simulink model "phase1_baseline"  (R2026a)
settings: Solver=VariableStepAuto
model workspace (MAT data in the model file):
  tau = 0
undefined symbols (not defined in the file): actuationDelay_s, simulationParams
settings Model: Creator=rayyu  LastModifiedBy=rayyu

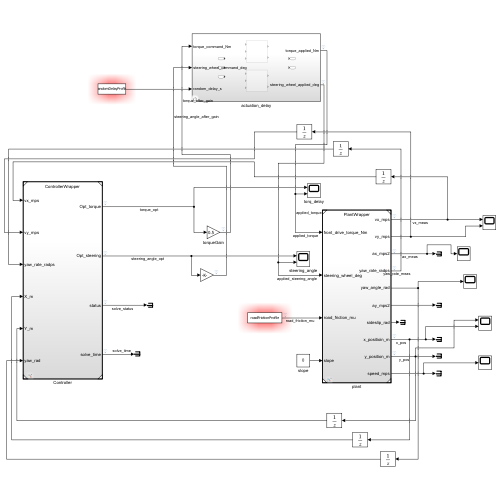
[thumbnail: Simulink's stored preview of the top-level diagram]
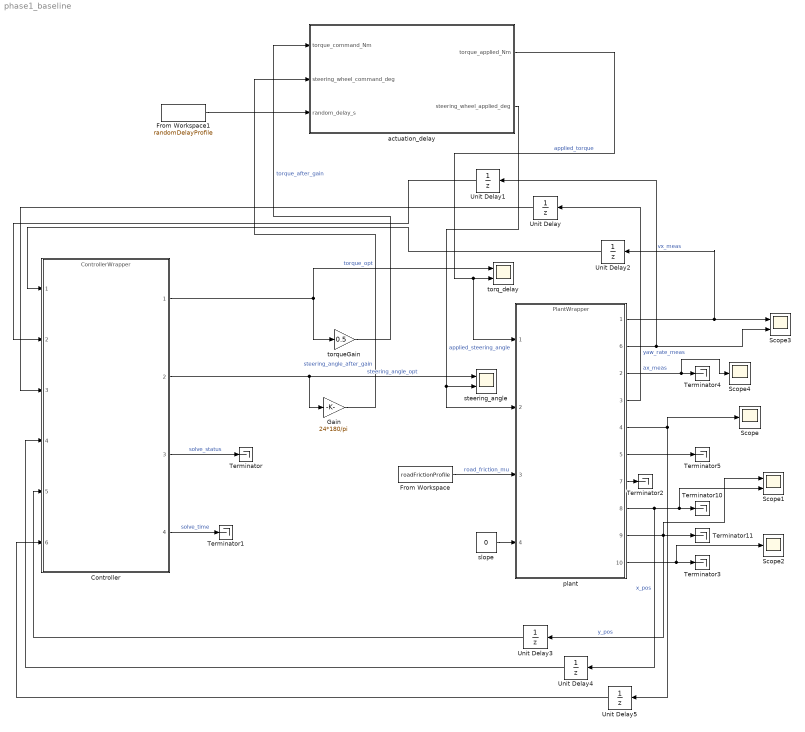
== system phase1_baseline ==
  Controller : ModelReference  ModelNameDialog=ControllerWrapper.slx  SimulationMode=Normal  ModelReferenceVersion=1.45
  From Workspace : FromWorkspace  VariableName=roadFrictionProfile  SampleTime=simulationParams.Ts_s  Interpolate=off  OutputAfterFinalValue=Holding final value
  From Workspace1 : FromWorkspace  VariableName=randomDelayProfile  Interpolate=off  OutputAfterFinalValue=Holding final value
  Gain : Gain  Gain=24*180/pi
  Scope : Scope
      settings: ActiveDisplayYMinimum=-1  ActiveDisplayYMaximum=1  DataLoggingVariableName=ScopeData4
  Scope1 : Scope  NumInputPorts=2
      settings: ActiveDisplayYMinimum=-21.988383930357102  ActiveDisplayYMaximum=153.74859051736982
  Scope2 : Scope
      settings: ActiveDisplayYMinimum=0  ActiveDisplayYMaximum=2.8635963178323579E-22  DataLoggingVariableName=ScopeData2
  Scope3 : Scope  NumInputPorts=2
      settings: ActiveDisplayYMinimum=-10.190231160058753  ActiveDisplayYMaximum=56.68780346222875  DataLoggingVariableName=ScopeData5
  Scope4 : Scope
      settings: ActiveDisplayYMinimum=-268098.75332313258  ActiveDisplayYMaximum=381760.8424542984  DataLoggingVariableName=ScopeData6
  Terminator{,1..5,10..11} (8 alike) : Terminator
  Unit Delay{,1..5} (6 alike) : UnitDelay  SampleTime=-1
  actuation_delay : Subsystem  Variant=on
  plant : ModelReference  ModelNameDialog=PlantWrapper.slx  SimulationMode=Normal  ModelReferenceVersion=1.23
      settings: PortSchema="{\"entries\":[{\"content\":{\"sides\":[{\"content\":{\"connectorIds\":[\"In1\",\"In2\",\"In3\",\"In4\"]},\"type\":\"ConnectorPlacement.EquallySpacedRectSide\",\"uuid\":\"bf665537-3fd8-4fa0-88a8-2cb308153754\"},{\"content\":{\"connectorIds\":[\"Out1\",\"Out6\",\"Out2\",\"Out3\",\"Out4\",\"Out5\",\"Out7\",\"Out8\",\"Out9\",\"Out10\"],\"side\":\"RIGHT\"},\"type\":\"ConnectorPlacement.EquallySpacedRectSide\",\"uuid\":\"a274990e-adc2-49b8-8679-a2f39e53ce6e\"},{\"content\":{\"side\":\"TOP\"},\"type\":\"ConnectorPlacement.EquallySpacedRectSide\",\"uuid\":\"963f9bff-e020-46b1-9958-cad0758083aa\"}]},\"type\":\"ConnectorPlacement.EquallySpacedConnector\",\"uuid\":\"fb8d0fca-1617-49ee-84dd-83e8b757a297\"}],\"packageUris\":[\"http://schema.mathworks.com/mf0/Connector/R2020b\"],\"version\":\"1.0\"}"
  slope : Constant  Value=0
  steering_angle : Scope  NumInputPorts=2
      settings: ActiveDisplayYMinimum=-183.84826338257844  ActiveDisplayYMaximum=186.50850743591388  DataLoggingVariableName=ScopeData3
  torq_delay : Scope  NumInputPorts=2
      settings: ActiveDisplayYMinimum=119.57395931342806  ActiveDisplayYMaximum=269.14536264631744  DataLoggingVariableName=ScopeData7
  torqueGain : Gain  Gain=0.5
  wires:
  plant/4 -> Unit Delay5/1, Scope/1
  plant/6 -> Unit Delay1/1, Scope3/2
  plant/1 -> Scope3/1, Unit Delay2/1  "vx_meas"
  plant/7 -> Terminator2/1
  slope/1 -> plant/4
  Controller/2 -> steering_angle/1, Gain/1  "steering_angle_opt"
  plant/3 -> Unit Delay/1  "yaw_rate_meas"
  plant/2 -> Scope4/1, Terminator4/1  "ax_meas"
  plant/10 -> Scope2/1, Terminator3/1
  From Workspace/1 -> plant/3  "road_friction_mu"
  Controller/3 -> Terminator/1  "solve_status"
  Controller/1 -> torqueGain/1, torq_delay/1  "torque_opt"
  Controller/4 -> Terminator1/1  "solve_time"
  plant/8 -> Unit Delay4/1, Scope1/2, Terminator10/1  "x_pos"
  plant/5 -> Terminator5/1
  Gain/1 -> actuation_delay/2(steering_wheel_command_deg)  "steering_angle_after_gain"
  plant/9 -> Unit Delay3/1, Scope1/1, Terminator11/1  "y_pos"
  Unit Delay/1 -> Controller/3
  Unit Delay1/1 -> Controller/2
  Unit Delay2/1 -> Controller/1
  Unit Delay3/1 -> Controller/5
  Unit Delay4/1 -> Controller/4
  Unit Delay5/1 -> Controller/6
  torqueGain/1 -> actuation_delay/1(torque_command_Nm)  "torque_after_gain"
  actuation_delay/1(torque_applied_Nm) -> plant/1, torq_delay/2  "applied_torque"
  actuation_delay/2(steering_wheel_applied_deg) -> plant/2, steering_angle/2  "applied_steering_angle"
  From Workspace1/1 -> actuation_delay/3(random_delay_s)

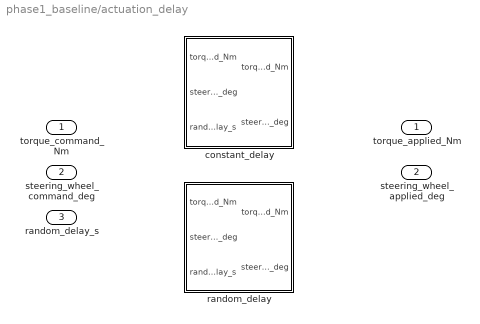
== system phase1_baseline/actuation_delay ==
  torque_command_Nm : Inport
  steering_wheel_command_deg : Inport  Port=2
  random_delay_s : Inport  Port=3
  constant_delay : Subsystem  VariantControl=delayMode == DELAY_MODE_CONSTANT
  random_delay : Subsystem  VariantControl=delayMode == DELAY_MODE_RANDOM
  torque_applied_Nm : Outport
  steering_wheel_applied_deg : Outport  Port=2

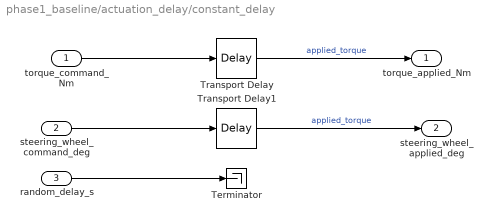
== system phase1_baseline/actuation_delay/constant_delay ==
  torque_command_Nm : Inport
  steering_wheel_command_deg : Inport  Port=2
  random_delay_s : Inport  Port=3
  Terminator : Terminator
  Transport Delay : TransportDelay  DelayTime=actuationDelay_s
  Transport Delay1 : TransportDelay  DelayTime=actuationDelay_s
  torque_applied_Nm : Outport
  steering_wheel_applied_deg : Outport  Port=2
  wires:
  torque_command_Nm/1 -> Transport Delay/1
  Transport Delay/1 -> torque_applied_Nm/1  "applied_torque"
  steering_wheel_command_deg/1 -> Transport Delay1/1
  Transport Delay1/1 -> steering_wheel_applied_deg/1  "applied_torque"
  random_delay_s/1 -> Terminator/1

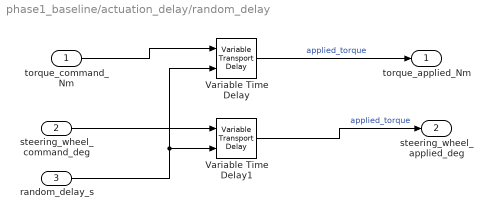
== system phase1_baseline/actuation_delay/random_delay ==
  torque_command_Nm : Inport
  steering_wheel_command_deg : Inport  Port=2
  random_delay_s : Inport  Port=3
  Variable Time Delay : VariableTransportDelay  MaximumDelay=maximumRandomDelay_s
  Variable Time Delay1 : VariableTransportDelay  MaximumDelay=maximumRandomDelay_s
  torque_applied_Nm : Outport
  steering_wheel_applied_deg : Outport  Port=2
  wires:
  Variable Time Delay1/1 -> steering_wheel_applied_deg/1  "applied_torque"
  torque_command_Nm/1 -> Variable Time Delay/1
  Variable Time Delay/1 -> torque_applied_Nm/1  "applied_torque"
  random_delay_s/1 -> Variable Time Delay/2, Variable Time Delay1/2
  steering_wheel_command_deg/1 -> Variable Time Delay1/1
